simulink subsystem "mixer"  (R2024b)
settings: Solver=VariableStepAuto  StartTime=0.0  StopTime=10.0  RelTol=1e-3
settings Model: Creator=thesa  LastModifiedBy=jack
settings RTWCC: GPUComputeCapability=3.5

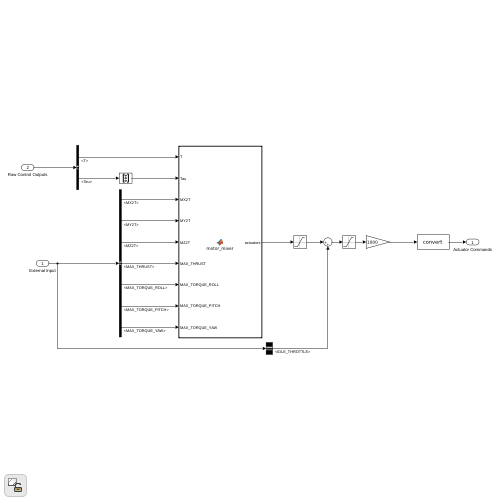
[thumbnail: Simulink's stored preview of the top-level diagram]
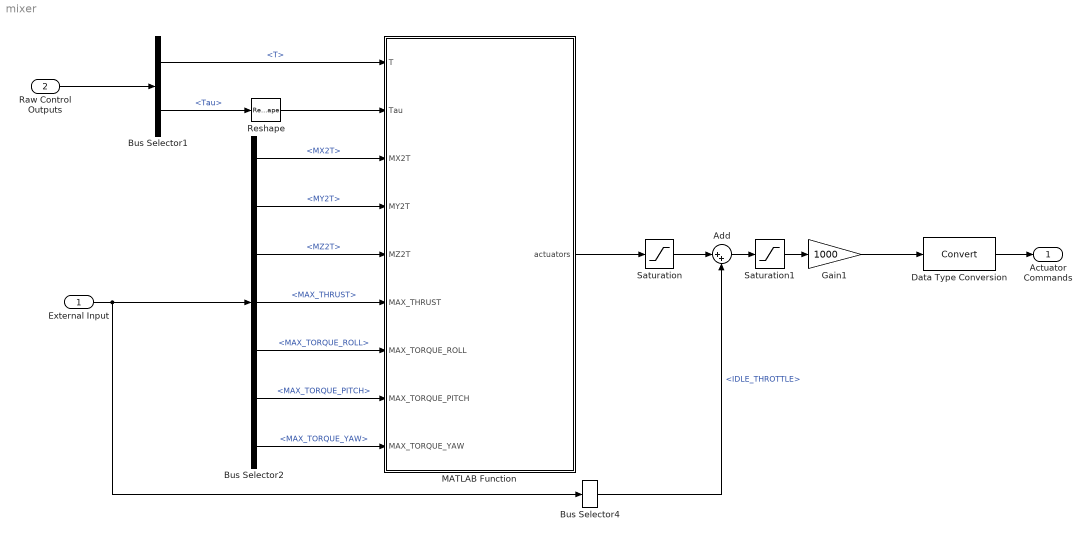
== system mixer ==
  External Input : Inport
  Raw Control Outputs : Inport  Port=2
  Add : Sum  Inputs=|++
  Bus Selector1 : BusSelector  OutputSignals=Control Outputs.T,Control Outputs.Tau
  Bus Selector2 : BusSelector  OutputSignals=Vehicle Parameters.MX2T,Vehicle Parameters.MY2T,Vehicle Parameters.MZ2T,Vehicle Parameters.MAX_THRUST,Vehicle Parameters.MAX_TORQUE_ROLL,Vehicle Parameters.MAX_TORQUE_PITCH,Vehicle Parameters.MAX_TORQUE_YAW
  Bus Selector4 : BusSelector  OutputSignals=Vehicle Parameters.IDLE_THROTTLE
  Data Type Conversion : DataTypeConversion  SaturateOnIntegerOverflow=off  RndMeth=Floor
  Gain1 : Gain  Gain=1000
  MATLAB Function : MATLAB Function  TreatAsAtomicUnit=on
  Reshape : Reshape  OutputDimensionality=Column vector (2-D)
  Saturation : Saturate  UpperLimit=1  LowerLimit=0
  Saturation1 : Saturate  UpperLimit=1  LowerLimit=0
  Actuator Commands : Outport
  wires:
  Bus Selector4/1 -> Add/2  "<IDLE_THROTTLE>"
  Saturation/1 -> Add/1
  Saturation1/1 -> Gain1/1
  MATLAB Function/1(actuators) -> Saturation/1
  Gain1/1 -> Data Type Conversion/1
  Add/1 -> Saturation1/1
  External Input/1 -> Bus Selector4/1, Bus Selector2/1
  Raw Control Outputs/1 -> Bus Selector1/1
  Bus Selector2/2 -> MATLAB Function/4(MY2T)  "<MY2T>"
  Bus Selector1/1 -> MATLAB Function/1(T)  "<T>"
  Bus Selector1/2 -> Reshape/1  "<Tau>"
  Bus Selector2/6 -> MATLAB Function/8(MAX_TORQUE_PITCH)  "<MAX_TORQUE_PITCH>"
  Bus Selector2/5 -> MATLAB Function/7(MAX_TORQUE_ROLL)  "<MAX_TORQUE_ROLL>"
  Bus Selector2/4 -> MATLAB Function/6(MAX_THRUST)  "<MAX_THRUST>"
  Bus Selector2/3 -> MATLAB Function/5(MZ2T)  "<MZ2T>"
  Bus Selector2/1 -> MATLAB Function/3(MX2T)  "<MX2T>"
  Bus Selector2/7 -> MATLAB Function/9(MAX_TORQUE_YAW)  "<MAX_TORQUE_YAW>"
  Reshape/1 -> MATLAB Function/2(Tau)
  Data Type Conversion/1 -> Actuator Commands/1

== matlab function mixer/MATLAB Function ==
  data: T input; actuators output; Tau input; MX2T input; MY2T input; MZ2T input; MAX_THRUST input; MAX_TORQUE_ROLL input; MAX_TORQUE_PITCH input; MAX_TORQUE_YAW input
function actuators  = motor_mixer(T, Tau, ...
    MX2T, MY2T, MZ2T, ...
    MAX_THRUST, MAX_TORQUE_ROLL, MAX_TORQUE_PITCH, MAX_TORQUE_YAW)

actuators  = motor_mixer(T, Tau, ...
    MX2T, MY2T, MZ2T, ...
    MAX_THRUST, MAX_TORQUE_ROLL, MAX_TORQUE_PITCH, MAX_TORQUE_YAW);

end
